simulink model "SelectionDepart_Numerique"  (R2023a)
settings: Solver=FixedStepDiscrete  StartTime=0.0  StopTime=0.05  RelTol=1e-3
values from neighbouring files (symbols this model uses):
  fba = 1.36*10^6-340*10^3-4*offseta    (= 888000)    [Code.m]
  fbn = (1.36*10^6)-(340*10^3)-offsetn    (= 930000)    [Code.m]
  m = 1    [Code.m]
  n = 0    [Code.m]
  offseta = 33*10^3    (= 33000)    [Code.m]
  offsetn = 90*10^3    (= 90000)    [Code.m]
  type = 0    [Code.m]
libraries: dspfdesign x11, dspsigops x1, dspsrcs4 x1
settings Model: Creator=roys2121  LastModifiedBy=jmoue
settings DebuggingCC: UnconnectedInputMsg=warning  UnconnectedOutputMsg=warning  UnconnectedLineMsg=warning
settings ModelReferenceCC: EnableRefExpFcnMdlSchedulingChecks=on
settings RTWCC: DLArmComputeVersion=19.05

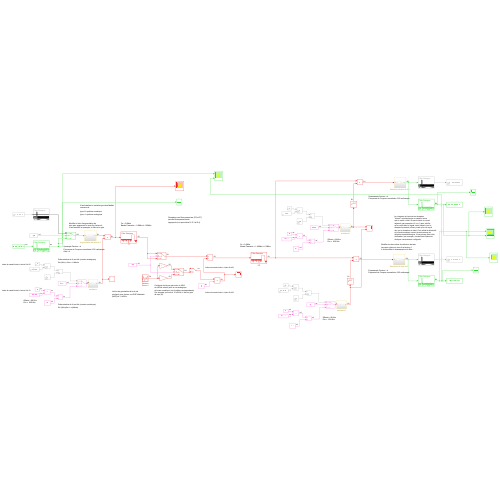
[thumbnail: Simulink's stored preview of the top-level diagram]
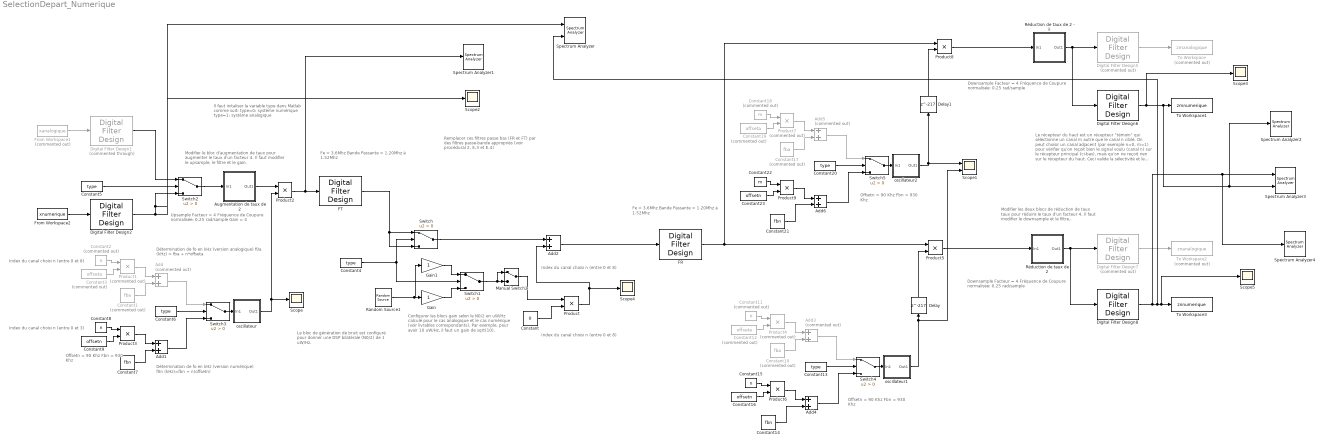
== system SelectionDepart_Numerique ==
  note: Upsample Facteur = 4
      | Fréquence de Coupure normalisée: 0.25 rad/sample
      | Gain = 4
  note: Le récepteur du haut est un récepteur
      | "témoin" qui sélectionne un canal m autre
      | que le canal n ciblé. On peut choisir un canal
      | adjacent (par exemple n=0, m=1) pour vérifier
      | qu'on reçoit bien le signal voulu (canal n) sur le
      | récepteur principal (ci-bas), mais qu'on ne reçoit
      | rien sur le récepteur du haut. Ceci valide la sélectivité
      | et le fonctionnement correct du mécanisme de
      | séleciton superhétérodyne. Vous pouvez faire cette
      | vérification, par exemple, via des blocs Spectrum
      | Analyzer correctement configurés.
  note: Modifier le bloc d'augmentation de
      | taux pour augmenter le taux d'un facteur 4.
      | Il faut modifier le upsample, le filtre et le gain.
  note: Remplacer ces filtres passe bas (FR et FT)
      | par des filtres passe-bande
      | appropriés (voir procédural 2, E.3 et E.4)
  note: Configurer les blocs gain selon le N0/2
      | en uW/Hz calculé pour le cas analogique
      | et le cas numérique (voir livrables correspondants).
      | Par exemple, pour avoir 10 uW/Hz, il faut un gain
      | de sqrt(10).
  note: Il faut initaliser la variable type dans Matlab
      | comme suit:
      |
      | type=0: système numérique
      | type=1: système analogique
  note: Le bloc de génération de bruit est
      | configuré pour donner une DSP bilatérale
      | (N0/2) de 1 uW/Hz.
  note: Index du canal choisi n (entre 0 et 8)
  note: Détermination de fo en kHz (version analogique)
      | f0a (kHz) = fba + n*offseta
  note: Détermination de fo en kHz (version numérique)
      | f0n (kHz)=fbn + n(offsetn)
  note: Index du canal choisi n (entre 0 et 3)
  note: Index du canal choisi n (entre 0 et 8)
  note: Index du canal choisi n (entre 0 et 8)
  note: Modifier les deux blocs de réduction de taux
      | taux pour réduire le taux d'un facteur 4.
      | Il faut modifier le downsample et le filtre..
  note: Downsample Facteur = 4
      | Fréquence de Coupure normalisée: 0.25 rad/sample
  note: Downsample Facteur = 4
      | Fréquence de Coupure normalisée: 0.25 rad/sample
  note: Fe = 3.6Mhz
      | Bande Passante = 1.20Mhz à 1.52Mhz
  note: Fe = 3.6Mhz
      | Bande Passante = 1.20Mhz à 1.52Mhz
  note: Offsetn = 90 Khz
      | Fbn =  930 Khz
  note: Offsetn = 90 Khz
      | Fbn =  930 Khz
  note: Offsetn = 90 Khz
      | Fbn =  930 Khz
  Add : Sum  Commented=on
  Add{1..2,4,6} (4 alike) : Sum
  Add3 : Sum  Commented=on
  Add5 : Sum  Commented=on
  Augmentation de taux de 2 : Subsystem
  Constant : Constant  Value=0
  Constant1 : Constant  Commented=on  Value=fba
  Constant10 : Constant  Commented=on  Value=fba
  Constant11 : Constant  Commented=on  Value=n
  Constant12 : Constant  Commented=on  Value=offseta
  Constant{4..6,13,20} (5 alike) : Constant  Value=type
  Constant14 : Constant  Value=fbn
  Constant15 : Constant  Value=n
  Constant16 : Constant  Value=offsetn
  Constant17 : Constant  Commented=on  Value=fba
  Constant18 : Constant  Commented=on  Value=m
  Constant19 : Constant  Commented=on  Value=offseta
  Constant2 : Constant  Commented=on  Value=n
  Constant21 : Constant  Value=fbn
  Constant22 : Constant  Value=m
  Constant23 : Constant  Value=offsetn
  Constant3 : Constant  Commented=on  Value=offseta
  Constant7 : Constant  Value=fbn
  Constant8 : Constant  Value=n
  Constant9 : Constant  Value=offsetn
  Delay : Delay  DelayLength=217  InitialCondition=0
  Delay1 : Delay  DelayLength=217  InitialCondition=0
  Digital Filter Design1 : dspfdesign/Digital Filter Design  Commented=through  mwdsp_browser_bugfix_var=off
  Digital Filter Design2 : dspfdesign/Digital Filter Design  mwdsp_browser_bugfix_var=off
  Digital Filter Design5 : dspfdesign/Digital Filter Design  Commented=on  mwdsp_browser_bugfix_var=off
  Digital Filter Design6 : dspfdesign/Digital Filter Design  mwdsp_browser_bugfix_var=off
  Digital Filter Design7 : dspfdesign/Digital Filter Design  Commented=on  mwdsp_browser_bugfix_var=off
  Digital Filter Design8 : dspfdesign/Digital Filter Design  mwdsp_browser_bugfix_var=off
  FR : dspfdesign/Digital Filter Design  mwdsp_browser_bugfix_var=off
  FT : dspfdesign/Digital Filter Design  mwdsp_browser_bugfix_var=off
  From Workspace1 : FromWorkspace  Commented=on  VariableName=xanalogique  SampleTime=1/3.2e6  Interpolate=off  ZeroCross=off  OutputAfterFinalValue=Setting to zero
  From Workspace2 : FromWorkspace  VariableName=xnumerique  SampleTime=1/3.2e6  Interpolate=off  OutputAfterFinalValue=Setting to zero
  Gain : Gain
  Gain1 : Gain
  Manual Switch2 : ManualSwitch
  Product{,2..3,5..6,8..9} (7 alike) : Product
  Product1 : Product  Commented=on
  Product4 : Product  Commented=on
  Product7 : Product  Commented=on
  Random Source1 : dspsrcs4/Random Source  SrcType=Gaussian  NormMethod=Ziggurat  CltLength=12  MinVal=0  MaxVal=1  MeanVal=0  VarVal=12.8  RepMode=Not repeatable  rawSeed=1  IsInherit=off  SampMode=Discrete  SampTime=1/12.8e6  SampFrame=1  DataType=Double  OutComplex=Real  OutputFrames=off
  Réduction de taux de 2 : Subsystem
  Réduction de taux de 2 - ii : Subsystem
  Scope{,2..5} (5 alike) : Scope
  Scope1 : Scope  NumInputPorts=2
  Spectrum Analyzer : SpectrumAnalyzer  NumInputPorts=2  WindowPosition=[1.000000,49.000000,1536.000000,793.000000,]  ScopeFrameLocation=window  SpectrumType=Power density  Span=3199999.9999999995  StartFrequency=-1599999.9999999998  StopFrequency=1599999.9999999998  SpectrumUnits=dBm/Hz  YLimits=[-353.1193091,31.24292564]  ColorLimits=[-80 20]  ShowLegend=on
      settings: OpenAtSimulationStart=off
  Spectrum Analyzer1 : SpectrumAnalyzer  WindowPosition=[263.000000,-47.000000,859.000000,793.000000,]  ScopeFrameLocation=window  SpectrumType=Power density  Span=3199999.9999999995  StartFrequency=-1599999.9999999998  StopFrequency=1599999.9999999998  SpectrumUnits=dBm/Hz  YLimits=[-221.78881257,0.57252366]  ColorLimits=[-80 20]  ShowLegend=on  ExpandToolstrip=on
      settings: OpenAtSimulationStart=off
  Spectrum Analyzer2 : SpectrumAnalyzer  WindowPosition=[452.000000,4.000000,859.000000,793.000000,]  ScopeFrameLocation=window  SpectrumType=Power density  Span=3199999.9999999995  StartFrequency=-1599999.9999999998  StopFrequency=1599999.9999999998  SpectrumUnits=dBm/Hz  YLimits=[-332.31238855,-110.52438926]  ColorLimits=[-80 20]  ShowLegend=on  ExpandToolstrip=on
      settings: OpenAtSimulationStart=off
  Spectrum Analyzer3 : SpectrumAnalyzer  NumInputPorts=2  WindowPosition=[1.000000,49.000000,1536.000000,793.000000,]  ScopeFrameLocation=window  SpectrumType=Power density  Span=3199999.9999999995  StartFrequency=-1599999.9999999998  StopFrequency=1599999.9999999998  SpectrumUnits=dBm/Hz  YLimits=[-337.43057268,-109.95570214]  ColorLimits=[-80 20]  ShowLegend=on
      settings: OpenAtSimulationStart=off
  Spectrum Analyzer4 : SpectrumAnalyzer  WindowPosition=[1.000000,49.000000,1536.000000,793.000000,]  ScopeFrameLocation=window  SpectrumType=Power density  Span=3199999.9999999995  StartFrequency=-1599999.9999999998  StopFrequency=1599999.9999999998  SpectrumUnits=dBm/Hz  YLimits=[-336.15497606,-121.43607168]  ColorLimits=[-80 20]  ShowLegend=on  ExpandToolstrip=on
      settings: OpenAtSimulationStart=off
  Switch{,1..5} (6 alike) : Switch  Criteria=u2 > Threshold  SaturateOnIntegerOverflow=off  InputSameDT=off
  To Workspace : ToWorkspace  Commented=on  VariableName=zmanalogique  SampleTime=-1
      settings: Save2DSignal=2-D array (concatenate along first dimension)
  To Workspace1 : ToWorkspace  VariableName=zmnumerique  SampleTime=-1
      settings: Save2DSignal=2-D array (concatenate along first dimension)
  To Workspace2 : ToWorkspace  Commented=on  VariableName=znanalogique  SampleTime=-1
      settings: Save2DSignal=2-D array (concatenate along first dimension)
  To Workspace3 : ToWorkspace  VariableName=znnumerique  SampleTime=-1
      settings: Save2DSignal=2-D array (concatenate along first dimension)
  oscillateur : Subsystem
  oscillateur1 : Subsystem
  oscillateur2 : Subsystem
  wires:
  From Workspace1/1 -> Digital Filter Design1/1
  From Workspace2/1 -> Digital Filter Design2/1
  oscillateur/1(Out1) -> Product2/2, Scope/1
  Constant2/1 -> Product1/1
  Constant3/1 -> Product1/2
  Constant1/1 -> Add/2
  Product1/1 -> Add/1
  Switch/1 -> Add2/1
  FT/1 -> Switch/3, Switch/1
  Constant4/1 -> Switch/2, Switch1/2
  Switch1/1 -> Manual Switch2/1, Manual Switch2/2
  Random Source1/1 -> Gain1/1, Gain/1
  Gain/1 -> Switch1/3
  Gain1/1 -> Switch1/1
  Augmentation de taux de 2/1(Out1) -> Product2/1
  Digital Filter Design2/1 -> Scope2/1, Spectrum Analyzer/1, Switch2/3
  Digital Filter Design1/1 -> Switch2/1
  Switch2/1 -> Augmentation de taux de 2/1(In1)
  Constant5/1 -> Switch2/2
  Constant6/1 -> Switch3/2
  Switch3/1 -> oscillateur/1(In1)
  Add/1 -> Switch3/1
  Constant8/1 -> Product3/1
  Constant9/1 -> Product3/2
  Constant7/1 -> Add1/2
  Product3/1 -> Add1/1
  Add1/1 -> Switch3/3
  Add2/1 -> FR/1
  Constant11/1 -> Product4/1
  Constant15/1 -> Product6/1
  Constant12/1 -> Product4/2
  Product4/1 -> Add3/1
  oscillateur1/1(Out1) -> Scope1/2, Delay/1
  Constant16/1 -> Product6/2
  Constant13/1 -> Switch4/2
  Add4/1 -> Switch4/3
  Constant14/1 -> Add4/2
  Constant10/1 -> Add3/2
  Add3/1 -> Switch4/1
  Product6/1 -> Add4/1
  Switch4/1 -> oscillateur1/1(In1)
  FR/1 -> Product8/1, Product5/1
  Delay/1 -> Product5/2
  Product9/1 -> Add6/1
  Add5/1 -> Switch5/1
  Delay1/1 -> Product8/2
  Constant21/1 -> Add6/2
  Constant19/1 -> Product7/2
  Add6/1 -> Switch5/3
  Switch5/1 -> oscillateur2/1(In1)
  Constant23/1 -> Product9/2
  Product7/1 -> Add5/1
  oscillateur2/1(Out1) -> Scope1/1, Delay1/1
  Constant20/1 -> Switch5/2
  Constant17/1 -> Add5/2
  Constant18/1 -> Product7/1
  Constant22/1 -> Product9/1
  Réduction de taux de 2 - ii/1(Out1) -> Digital Filter Design6/1, Digital Filter Design5/1
  Réduction de taux de 2/1(Out1) -> Digital Filter Design8/1, Digital Filter Design7/1
  Digital Filter Design7/1 -> To Workspace2/1
  Digital Filter Design8/1 -> Spectrum Analyzer4/1, Spectrum Analyzer3/1, Spectrum Analyzer/2, Scope5/1, To Workspace3/1
  Digital Filter Design5/1 -> To Workspace/1
  Digital Filter Design6/1 -> Scope3/1, Spectrum Analyzer2/1, Spectrum Analyzer3/2, To Workspace1/1
  Product8/1 -> Réduction de taux de 2 - ii/1(In1)
  Product5/1 -> Réduction de taux de 2/1(In1)
  Product2/1 -> Spectrum Analyzer1/1, FT/1
  Product/1 -> Scope4/1, Add2/2
  Manual Switch2/1 -> Product/1
  Constant/1 -> Product/2

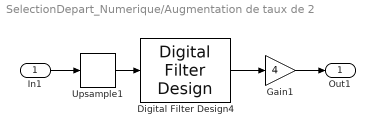
== system SelectionDepart_Numerique/Augmentation de taux de 2 ==
  In1 : Inport
  Digital Filter Design4 : dspfdesign/Digital Filter Design  mwdsp_browser_bugfix_var=off
  Gain1 : Gain  Gain=4
  Upsample1 : dspsigops/Upsample  FactorSource=Dialog parameter  N=4  Nmax=16  phase=0  RateOptions=Allow multirate processing  ic=0  mode=Unused parameter value
  Out1 : Outport
  wires:
  Upsample1/1 -> Digital Filter Design4/1
  Gain1/1 -> Out1/1
  Digital Filter Design4/1 -> Gain1/1
  In1/1 -> Upsample1/1

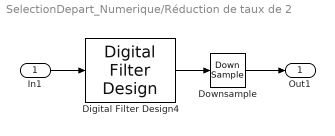
== system SelectionDepart_Numerique/Réduction de taux de 2 ==
  In1 : Inport
  Digital Filter Design4 : dspfdesign/Digital Filter Design  mwdsp_browser_bugfix_var=off
  Downsample : DownSample  N=4  RateOptions=Allow multirate processing
  Out1 : Outport
  wires:
  In1/1 -> Digital Filter Design4/1
  Digital Filter Design4/1 -> Downsample/1
  Downsample/1 -> Out1/1

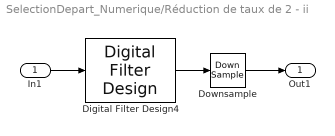
== system SelectionDepart_Numerique/Réduction de taux de 2 - ii ==
  In1 : Inport
  Digital Filter Design4 : dspfdesign/Digital Filter Design  mwdsp_browser_bugfix_var=off
  Downsample : DownSample  N=4  RateOptions=Allow multirate processing
  Out1 : Outport
  wires:
  Downsample/1 -> Out1/1
  In1/1 -> Digital Filter Design4/1
  Digital Filter Design4/1 -> Downsample/1

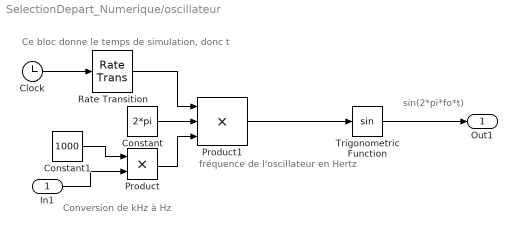
== system SelectionDepart_Numerique/oscillateur ==
  note: sin(2*pi*fo*t)
  note: Conversion de kHz à Hz
  note: Ce bloc donne le temps de simulation, donc t
  note: fréquence de l'oscillateur en Hertz
  In1 : Inport
  Clock : Clock
  Constant : Constant  Value=2*pi
  Constant1 : Constant  Value=1000
  Product : Product
  Product1 : Product  Inputs=3
  Rate Transition : RateTransition  OutPortSampleTime=1/12.8e6
  Trigonometric Function : Trigonometry
  Out1 : Outport
  wires:
  Trigonometric Function/1 -> Out1/1
  Product1/1 -> Trigonometric Function/1
  Constant/1 -> Product1/2
  Product/1 -> Product1/3
  In1/1 -> Product/2
  Constant1/1 -> Product/1
  Clock/1 -> Rate Transition/1
  Rate Transition/1 -> Product1/1

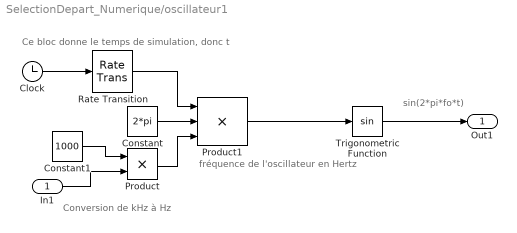
== system SelectionDepart_Numerique/oscillateur1 ==
  note: sin(2*pi*fo*t)
  note: Conversion de kHz à Hz
  note: Ce bloc donne le temps de simulation, donc t
  note: fréquence de l'oscillateur en Hertz
  In1 : Inport
  Clock : Clock
  Constant : Constant  Value=2*pi
  Constant1 : Constant  Value=1000
  Product : Product
  Product1 : Product  Inputs=3
  Rate Transition : RateTransition  OutPortSampleTime=1/12.8e6
  Trigonometric Function : Trigonometry
  Out1 : Outport
  wires:
  Trigonometric Function/1 -> Out1/1
  Product1/1 -> Trigonometric Function/1
  Constant/1 -> Product1/2
  Product/1 -> Product1/3
  In1/1 -> Product/2
  Constant1/1 -> Product/1
  Clock/1 -> Rate Transition/1
  Rate Transition/1 -> Product1/1

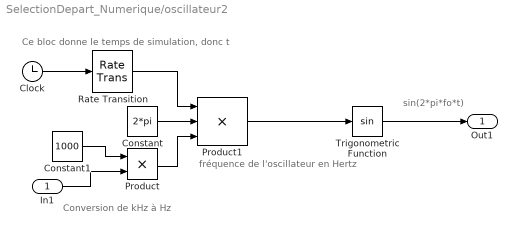
== system SelectionDepart_Numerique/oscillateur2 ==
  note: sin(2*pi*fo*t)
  note: Conversion de kHz à Hz
  note: Ce bloc donne le temps de simulation, donc t
  note: fréquence de l'oscillateur en Hertz
  In1 : Inport
  Clock : Clock
  Constant : Constant  Value=2*pi
  Constant1 : Constant  Value=1000
  Product : Product
  Product1 : Product  Inputs=3
  Rate Transition : RateTransition  OutPortSampleTime=1/12.8e6
  Trigonometric Function : Trigonometry
  Out1 : Outport
  wires:
  Trigonometric Function/1 -> Out1/1
  Product1/1 -> Trigonometric Function/1
  Constant/1 -> Product1/2
  Product/1 -> Product1/3
  In1/1 -> Product/2
  Constant1/1 -> Product/1
  Clock/1 -> Rate Transition/1
  Rate Transition/1 -> Product1/1
